simulink model "inverted_pendulum_linear_simulation"  (R2018a)
settings: Solver=VariableStepAuto  StartTime=0.0  StopTime=5  RelTol=1e-3
values from neighbouring files (symbols this model uses):
  A = [0          1       0;     g/l_cm      0       c_e*c_m/(J_p*R_a);     -g/l_cm     0       -c_m*c_e/(J_w*R_a)]    [pendulum_parameters.m]
  B = [0;     -c_m/(J_p*R_a);     c_m/(J_w*R_a)]    [pendulum_parameters.m]
  Kr = -Kr    [pendulum_parameters.m]
  MAX_U = 18    [pendulum_parameters.m]
  Ts = 50e-3    (= 0.05)    [pendulum_parameters.m]
settings Model: Creator=Gospar  LastModifiedBy=Gospar

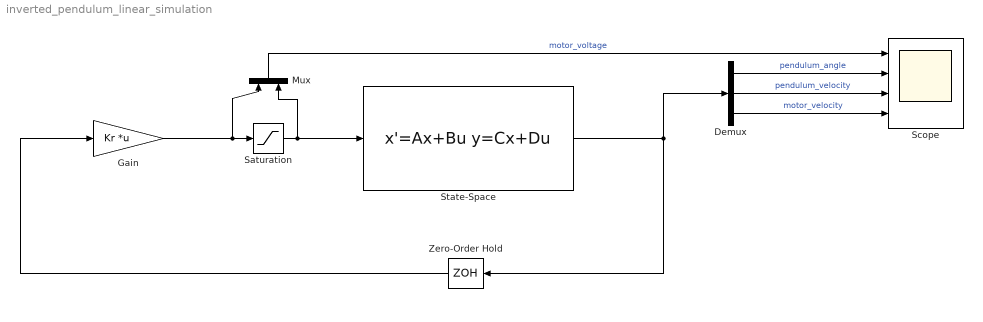
== system inverted_pendulum_linear_simulation ==
  Demux : Demux  Outputs=3
  Gain : Gain  Gain=Kr  Multiplication=Matrix(K*u)
  Mux : Mux  Inputs=2
  Saturation : Saturate  UpperLimit=MAX_U  LowerLimit=-MAX_U
  Scope : Scope  NumInputPorts=4
  State-Space : StateSpace  A=A  B=B  C=eye(3)  D=[0;0;0]  InitialCondition=[5*pi/180 0 0]
  Zero-Order Hold : ZeroOrderHold  SampleTime=Ts
  wires:
  Zero-Order Hold/1 -> Gain/1
  State-Space/1 -> Demux/1, Zero-Order Hold/1
  Saturation/1 -> State-Space/1, Mux/2
  Gain/1 -> Mux/1, Saturation/1
  Mux/1 -> Scope/1  "motor_voltage"
  Demux/1 -> Scope/2  "pendulum_angle"
  Demux/2 -> Scope/3  "pendulum_velocity"
  Demux/3 -> Scope/4  "motor_velocity"
